simulink model "Lab1_parameter_estimation_student"  (R2024b)
settings: Solver=FixedStepAuto  StartTime=0.0  StopTime=inf  FixedStep=0.001  RelTol=1e-3
values from neighbouring files (symbols this model uses):
  motor_B = 0.0001    [Lab1_motor_params_student.m]
  motor_Eff = 0.5    [Lab1_motor_params_student.m]
  motor_J = 0.001    [Lab1_motor_params_student.m]
  motor_Ke = 0.05    [Lab1_motor_params_student.m]
  motor_L = 0.01    [Lab1_motor_params_student.m]
  motor_R = 1.00    (= 1)    [Lab1_motor_params_student.m]
libraries: simulink x1
settings Model: Creator=tanawatp  LastModifiedBy=User
settings RTWCC: GPUComputeCapability=3.5

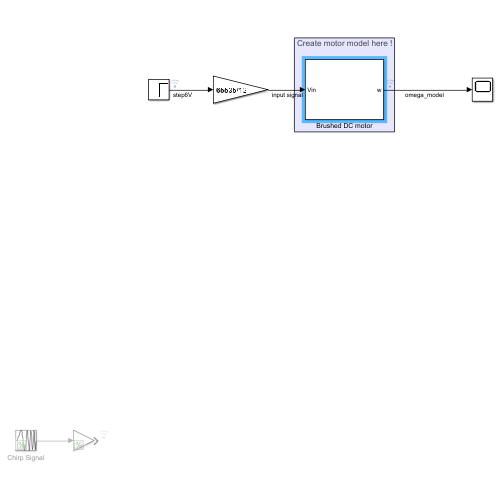
[thumbnail: Simulink's stored preview of the top-level diagram]
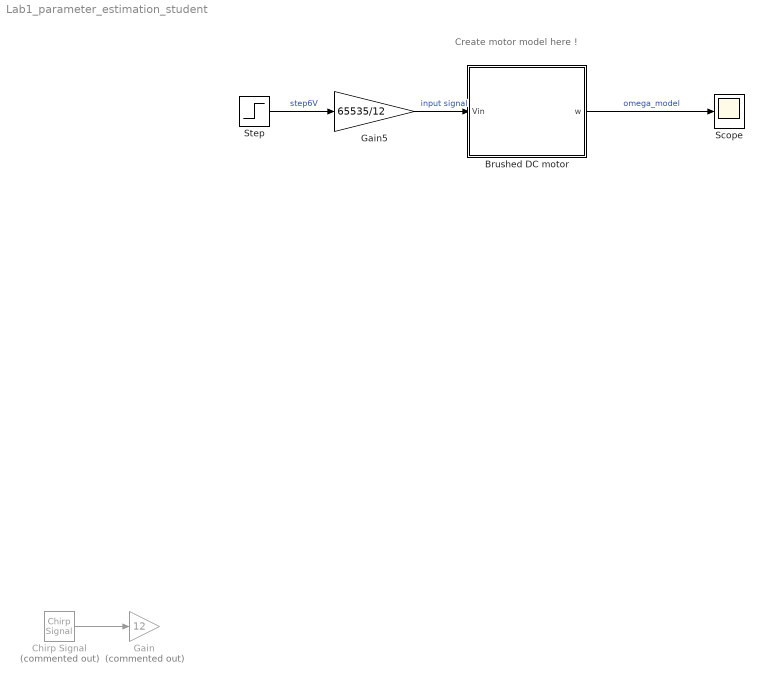
== system Lab1_parameter_estimation_student ==
  note: Create motor model here !
  Brushed DC motor : Subsystem
  Chirp Signal : simulink/Sources/Chirp Signal  Commented=on  f1=0.1  T=40  f2=5
  Gain : Gain  Commented=on  Gain=12
  Gain5 : Gain  Gain=65535/12
  Scope : Scope
  Step : Step  After=12  SampleTime=0
  wires:
  Brushed DC motor/1(w) -> Scope/1  "omega_model"
  Chirp Signal/1 -> Gain/1
  Gain5/1 -> Brushed DC motor/1(Vin)  "input signal"
  Step/1 -> Gain5/1  "step6V"

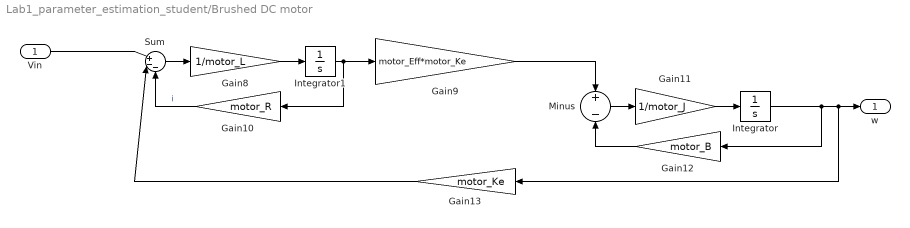
== system Lab1_parameter_estimation_student/Brushed DC motor ==
  Vin : Inport
  Gain10 : Gain  Gain=motor_R
  Gain11 : Gain  Gain=1/motor_J
  Gain12 : Gain  Gain=motor_B
  Gain13 : Gain  Gain=motor_Ke
  Gain8 : Gain  Gain=1/motor_L
  Gain9 : Gain  Gain=motor_Eff*motor_Ke
  Integrator : Integrator
  Integrator1 : Integrator
  Minus : Sum  Inputs=+-
  Sum : Sum  Inputs=|+--
  w : Outport
  wires:
  Vin/1 -> Sum/1
  Sum/1 -> Gain8/1
  Integrator1/1 -> Gain9/1, Gain10/1
  Gain8/1 -> Integrator1/1
  Gain10/1 -> Sum/3  "i"
  Gain9/1 -> Minus/1
  Integrator/1 -> Gain13/1, w/1, Gain12/1
  Gain12/1 -> Minus/2
  Minus/1 -> Gain11/1
  Gain11/1 -> Integrator/1
  Gain13/1 -> Sum/2
